simulink model "Transfomer_"  (R2020a)
settings: Solver=VariableStepAuto  StartTime=0.0  StopTime=0.1  RelTol=1e-3
undefined symbols (not defined in the file or in its folder): D1, Delta
libraries: powerlib x24
settings Model: Creator=JAYANT JETHI  LastModifiedBy=chait
settings SFSimCC: CustomCodeUndefinedFunction=UseInterfaceOnly

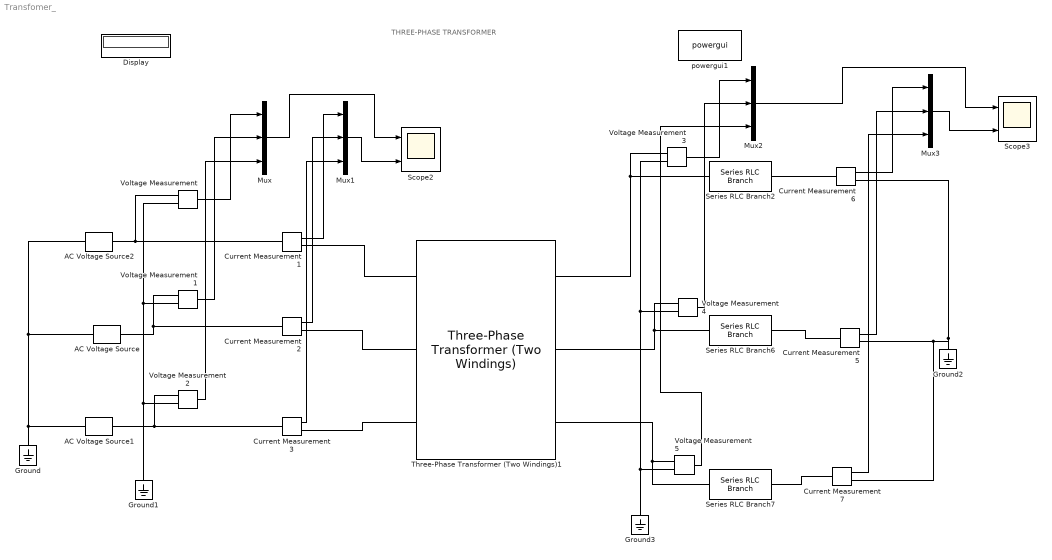
== system Transfomer_ ==
  note: THREE-PHASE TRANSFORMER
  AC Voltage Source : powerlib/Electrical Sources/AC Voltage Source  Amplitude=440  Phase=120  Frequency=50  SampleTime=0  Measurements=None  BusType=swing  Pref=10e3  Qref=0  Qmin=-inf  Qmax=+inf
  AC Voltage Source1 : powerlib/Electrical Sources/AC Voltage Source  Amplitude=440  Phase=-120  Frequency=50  SampleTime=0  Measurements=None  BusType=swing  Pref=10e3  Qref=0  Qmin=-inf  Qmax=+inf
  AC Voltage Source2 : powerlib/Electrical Sources/AC Voltage Source  Amplitude=440  Phase=0  Frequency=50  SampleTime=0  Measurements=None  BusType=swing  Pref=10e3  Qref=0  Qmin=-inf  Qmax=+inf
  Current Measurement{1..3,5..7} (6 alike) : powerlib/Measurements/Current Measurement  PhasorSimulation=off  OutputType=Complex  PSBequivalent=0
  Display : Display
  Ground{,1..3} (4 alike) : powerlib/Elements/Ground  LConnTagsString=a
  Mux{,1..3} (4 alike) : Mux  Inputs=3
  Scope2 : Scope  NumInputPorts=2
  Scope3 : Scope  NumInputPorts=2
  Series RLC Branch2 : powerlib/Elements/Series RLC Branch  LConnTagsString=__new0  RConnTagsString=__new0  BranchType=R  Resistance=220  Inductance=1e-3  SetiL0=off  InitialCurrent=0  Capacitance=1e-6  Setx0=off  InitialVoltage=0  Measurements=None
  Series RLC Branch6 : powerlib/Elements/Series RLC Branch  LConnTagsString=__new0  RConnTagsString=__new0  BranchType=R  Resistance=220  Inductance=1e-3  SetiL0=off  InitialCurrent=0  Capacitance=1e-6  Setx0=off  InitialVoltage=0  Measurements=None
  Series RLC Branch7 : powerlib/Elements/Series RLC Branch  LConnTagsString=__new0  RConnTagsString=__new0  BranchType=R  Resistance=220  Inductance=1e-3  SetiL0=off  InitialCurrent=0  Capacitance=1e-6  Setx0=off  InitialVoltage=0  Measurements=None
  Three-Phase Transformer (Two Windings)1 : powerlib/Elements/Three-Phase Transformer (Two Windings)  Winding1Connection=Delta (D1)  Winding2Connection=Yg  CoreType=Three single-phase transformers  SetSaturation=off  Hysteresis=off  DataFile='hysteresis'  SetInitialFlux=off  Measurements=None  UNITS=pu  NominalPower=[ 250e6 , 60 ]  Winding1=[ 440e3 , 0.002 , 0.08 ]  Winding2=[ 315e3 , 0.002 , 0.08 ]  Rm=500  Lm=500  L0=0.5  Saturation=[ 0,0 ; 0.0024,1.2 ; 1.0,1.52 ]  InitialFluxes=[ 0.8 , -0.8 , 0.7 ]  BreakLoop=off  DiscreteSolver=Trapezoidal iterative  DataType=off  TransfoNumber=1
  Voltage Measurement{,1..5} (6 alike) : powerlib/Measurements/Voltage Measurement  PhasorSimulation=off  OutputType=Complex  PSBequivalent=0
  powergui1 : powerlib/powergui  Priority=1  SimulationMode=Continuous  SampleTime=50e-6  frequency=60  Iterations=50  frequencyindice=50  Pbase=100e6  ErrMax=1e-4  UnitsV=kV  UnitsW=MW  buscounter=0  FunctionMessages=off  echomessages=off  EnableUseOfTLC=off  CurrentSourceSwitches=off  DisableSnubberDevices=off  DisableRonSwitches=off  DisableVfSwitches=off  DisplayEquations=off  AutomaticDiscreteSolvers=off  SolverType=Tustin/Backward Euler (TBE)  Interpol=off  ExternalGateDelay=off  methode=off  Ts=100  x0status=blocks  SPID=on  SwTol=0  HookPort=off  NonlinearTolerance=0  nMaxIteration=15  ContinueOnMaxIteration=off  RestoreLinks=warning  ResistiveCurrentMeasurement=off  Frange=[0:2:500]  Ylog=off  Xlog=on  ShowGrid=off  save=off  variable=ZData  structure=0  ZoomFFT=off  StartTime=0.0  cycles=1  DisplayStyle=1  fundamental=60  FreqAxis=off  MaxFrequency=1000  frequencyindicesteady=1  RmsSteady=1  display=off
  wires:
  Voltage Measurement/1 -> Mux/1
  Voltage Measurement1/1 -> Mux/2
  Voltage Measurement2/1 -> Mux/3
  Current Measurement1/1 -> Mux1/1
  Current Measurement2/1 -> Mux1/2
  Current Measurement3/1 -> Mux1/3
  Mux/1 -> Scope2/1
  Mux1/1 -> Scope2/2
  Voltage Measurement3/1 -> Mux2/1
  Voltage Measurement4/1 -> Mux2/2
  Voltage Measurement5/1 -> Mux2/3
  Mux2/1 -> Scope3/1
  Mux3/1 -> Scope3/2
  Current Measurement6/1 -> Mux3/1
  Current Measurement5/1 -> Mux3/2
  Current Measurement7/1 -> Mux3/3
  connections:
  Ground/LConn1 -- AC Voltage Source2/LConn1 -- AC Voltage Source/LConn1 -- AC Voltage Source1/LConn1
  AC Voltage Source2/RConn1 -- Current Measurement1/LConn1 -- Voltage Measurement/LConn1
  AC Voltage Source/RConn1 -- Current Measurement2/LConn1 -- Voltage Measurement1/LConn1
  AC Voltage Source1/RConn1 -- Current Measurement3/LConn1 -- Voltage Measurement2/LConn1
  Voltage Measurement/LConn2 -- Voltage Measurement1/LConn2 -- Ground1/LConn1 -- Voltage Measurement2/LConn2
  Current Measurement2/RConn1 -- Three-Phase Transformer (Two Windings)1/LConn2
  Current Measurement3/RConn1 -- Three-Phase Transformer (Two Windings)1/LConn3
  Current Measurement1/RConn1 -- Three-Phase Transformer (Two Windings)1/LConn1
  Three-Phase Transformer (Two Windings)1/RConn2 -- Voltage Measurement4/LConn1 -- Series RLC Branch6/LConn1
  Series RLC Branch7/LConn1 -- Voltage Measurement5/LConn1 -- Three-Phase Transformer (Two Windings)1/RConn3
  Three-Phase Transformer (Two Windings)1/RConn1 -- Voltage Measurement3/LConn1 -- Series RLC Branch2/LConn1
  Current Measurement5/RConn1 -- Current Measurement7/RConn1 -- Current Measurement6/RConn1 -- Ground2/LConn1
  Series RLC Branch2/RConn1 -- Current Measurement6/LConn1
  Series RLC Branch6/RConn1 -- Current Measurement5/LConn1
  Series RLC Branch7/RConn1 -- Current Measurement7/LConn1
  Voltage Measurement3/LConn2 -- Voltage Measurement5/LConn2 -- Ground3/LConn1 -- Voltage Measurement4/LConn2
